simulink model "LinearADPSimullink_R2014b"  (R2014b)
settings: Solver=ode45  StartTime=0.0  StopTime=10  MaxStep=0.0001  RelTol=1e-3
undefined symbols (not defined in the file): rank
libraries: simulink x4
settings Model: Creator=Yuri  LastModifiedBy=yujiang
settings SolverCC: ZeroCrossControl=EnableAll  ZeroCrossAlgorithm=Adaptive
settings DebuggingCC: AlgebraicLoopMsg=none  MultiTaskDSMMsg=none  FrameProcessingCompatibilityMsg=error
settings RTWCC: GenCodeOnly=on

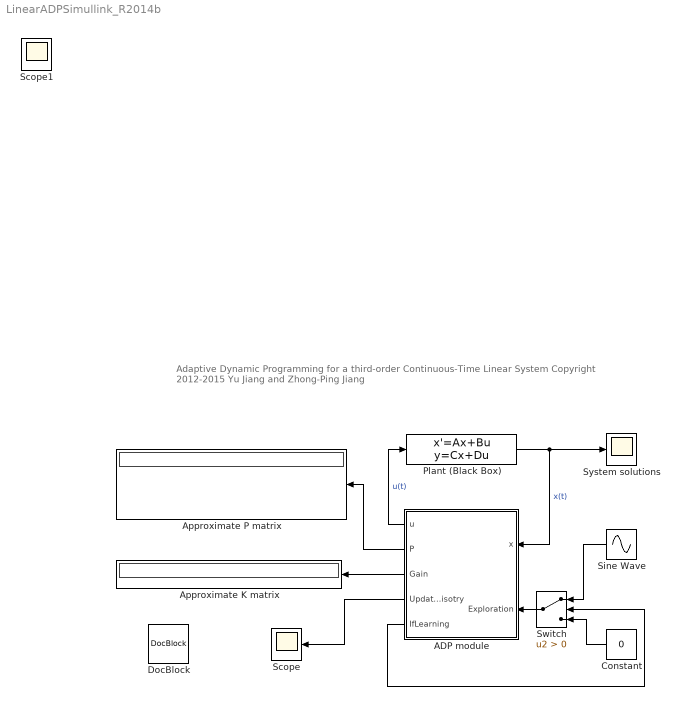
== system LinearADPSimullink_R2014b ==
  note: Adaptive Dynamic Programming for a third-order Continuous-Time Linear System
      |
      | Copyright 2012-2015 Yu Jiang and Zhong-Ping Jiang
  ADP module : Subsystem  mask{K=[0,0,0], Q=eye(3), R=1, dT=0.1, epsilon=.00005}
      mask prompts: K "Initial Gain K (e.g., [0,0])"; Q "Weight Matrix Q (e.g., eye(2))"; R "Weight R (e.g., 1)"; dT "Linearning Interval (e.g., 0.01)"; epsilon "Threshold (e.g., 0.00001)"
  Approximate K matrix : Display
  Approximate P matrix : Display
  Constant : Constant  Value=0
  DocBlock : simulink/Model-Wide Utilities/DocBlock  DocumentType=Text
      content=|
      | %To verify the results, try:
      |
      | A = [0 1 0; 0 0 1;-0.1 -0.5 -0.7];
      | B = [0;0;1];
      | Q = eye(3);
      | R = 1;
      |
      | [Popt,~,Kopt] = care(A,B,Q,R)
  Plant (Black Box) : StateSpace  A=[0 1 0; 0 0 1;-0.1 -0.5 -0.7]  B=[0;0;1]  C=eye(3)  D=zeros(3,1)  X0=[10;-10;15]
  Scope : Scope
      settings: SaveName=ScopeData2
  Sine Wave : Sin  Amplitude=2  Frequency=10  SampleTime=0.0001
  Switch : Switch  Criteria=u2 > Threshold  SampleTime=0.0001
  "System solutions " : Scope
      settings: ShowLegends=on  TimeRange=10  YMin=-10  YMax=20
  Scope1 : Scope
      settings: SaveName=ScopeData2
  wires:
  Plant (Black Box)/1 -> ADP module/1(x), "System solutions "/1  "x(t)"
  ADP module/1(u) -> Plant (Black Box)/1  "u(t)"
  ADP module/2("P ") -> Approximate P matrix/1
  ADP module/3(Gain) -> Approximate K matrix/1
  ADP module/4(UpdateHisotry) -> Scope/1
  Sine Wave/1 -> Switch/1
  Switch/1 -> ADP module/2(Exploration)
  ADP module/5(IfLearning) -> Switch/2
  Constant/1 -> Switch/3

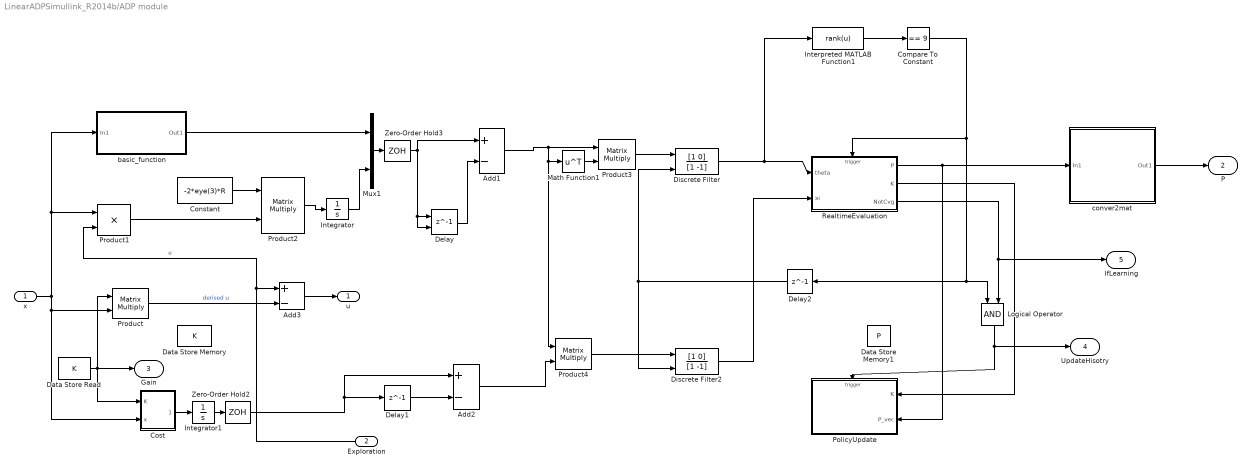
== system LinearADPSimullink_R2014b/ADP module ==
  x : Inport  PortDimensions=3
  Exploration : Inport  Port=2
  Add1 : Sum  Inputs=+-
  Add2 : Sum  Inputs=+-
  Add3 : Sum  Inputs=+-
  Compare To Constant : simulink/Logic and Bit Operations/Compare To Constant  relop===  const=9  OutDataTypeStr=boolean
  Constant : Constant  Value=-2*eye(3)*R  VectorParams1D=off
  Cost : Subsystem
  Data Store Memory : DataStoreMemory  Priority=1  DataStoreName=K  InitialValue=K  VectorParams1D=off  Dimensions=[1,3]
  Data Store Memory1 : DataStoreMemory  DataStoreName=P  InitialValue=-1*ones(6,1)
  Data Store Read : DataStoreRead  DataStoreName=K  SampleTime=0
  Delay : Delay  DelayLength=1  InitialConditionSource=Input port  InitialCondition=0  SampleTime=dT
      settings: InputPortMap=u0,p4
  Delay1 : Delay  DelayLength=1  InitialCondition=0  SampleTime=dT
  Delay2 : Delay  DelayLength=1  InitialCondition=0  SampleTime=dT
  Discrete Filter : DiscreteFilter  Numerator=[1 0]  Denominator=[1 -1]  ExternalReset=Rising  FilterStructure=Direct form I  SampleTime=dT  NumAccumDataTypeStr=Inherit: Same as product output  OutDataTypeStr=Inherit: Same as input
      settings: InputPortMap=u0,r7
  Discrete Filter2 : DiscreteFilter  Numerator=[1 0]  Denominator=[1 -1]  ExternalReset=Rising  FilterStructure=Direct form I  SampleTime=dT  NumAccumDataTypeStr=Inherit: Same as product output  OutDataTypeStr=Inherit: Same as input
      settings: InputPortMap=u0,r7
  Integrator : Integrator
  Integrator1 : Integrator
  Interpreted MATLAB Function1 : MATLABFcn  MATLABFcn=rank(u)  OutputDimensions=1
  Logical Operator : Logic  AllPortsSameDT=off  OutDataTypeStr=boolean
  Math Function1 : Math  Operator=transpose  SaturateOnIntegerOverflow=on
  Mux1 : Mux  Inputs=2
  PolicyUpdate : Subsystem
  Product{,2..4} (4 alike) : Product  Multiplication=Matrix(*)
  Product1 : Product
  RealtimeEvaluation : Subsystem
  Zero-Order Hold2 : ZeroOrderHold  SampleTime=dT
  Zero-Order Hold3 : ZeroOrderHold  SampleTime=dT
  basic_function : Subsystem
  conver2mat : Subsystem
  u : Outport
  "P " : Outport  Port=2
  Gain : Outport  Port=3
  UpdateHisotry : Outport  Port=4
  IfLearning : Outport  Port=5
  wires:
  RealtimeEvaluation/3(NotCvg) -> Logical Operator/2, IfLearning/1
  Exploration/1 -> Add3/1, Product1/2  "e"
  Logical Operator/1 -> PolicyUpdate/Trigger, UpdateHisotry/1
  Compare To Constant/1 -> Delay2/1, Logical Operator/1, RealtimeEvaluation/Trigger
  Add1/1 -> Product3/1, Math Function1/1, Product4/1
  Delay2/1 -> Discrete Filter2/2, Discrete Filter/2
  Zero-Order Hold2/1 -> Delay1/1, Add2/1
  Mux1/1 -> Zero-Order Hold3/1
  Discrete Filter2/1 -> RealtimeEvaluation/2(xi)
  Discrete Filter/1 -> Interpreted MATLAB Function1/1, RealtimeEvaluation/1(theta)
  Product4/1 -> Discrete Filter2/1
  Add2/1 -> Product4/2
  Product3/1 -> Discrete Filter/1
  Math Function1/1 -> Product3/2
  Add3/1 -> u/1
  Delay1/1 -> Add2/2
  Integrator1/1 -> Zero-Order Hold2/1
  Cost/1(r(x,uk)) -> Integrator1/1
  Delay/1 -> Add1/2
  Zero-Order Hold3/1 -> Add1/1, Delay/1, Delay/2
  Integrator/1 -> Mux1/2
  Product2/1 -> Integrator/1
  Constant/1 -> Product2/1
  Product1/1 -> Product2/2
  Data Store Read/1 -> Product/1, Cost/1(K), Gain/1
  Product/1 -> Add3/2  "derised u"
  x/1 -> basic_function/1(In1), Product1/1, Product/2, Cost/2(x)
  RealtimeEvaluation/1(P) -> PolicyUpdate/2("P_vec "), conver2mat/1(In1)
  RealtimeEvaluation/2(K) -> PolicyUpdate/1(K)
  Interpreted MATLAB Function1/1 -> Compare To Constant/1
  basic_function/1(Out1) -> Mux1/1
  conver2mat/1(Out1) -> "P "/1

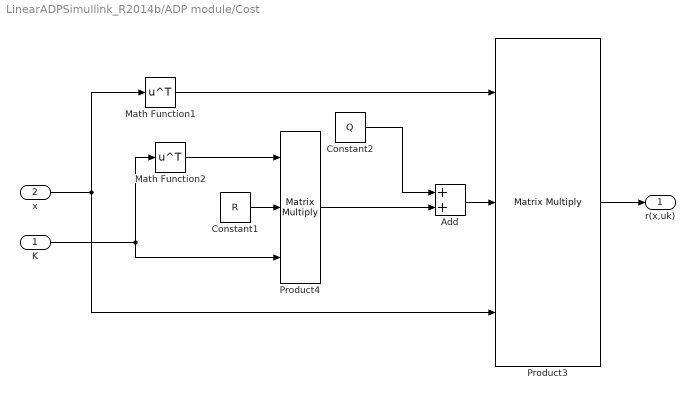
== system LinearADPSimullink_R2014b/ADP module/Cost ==
  K : Inport
  x : Inport  Port=2  PortDimensions=3
  Add : Sum
  Constant1 : Constant  Value=R
  Constant2 : Constant  Value=Q
  Math Function1 : Math  Operator=transpose  SaturateOnIntegerOverflow=on
  Math Function2 : Math  Operator=transpose  SaturateOnIntegerOverflow=on
  Product3 : Product  Inputs=3  Multiplication=Matrix(*)
  Product4 : Product  Inputs=3  Multiplication=Matrix(*)
  r(x,uk) : Outport
  wires:
  Math Function2/1 -> Product4/1
  Constant1/1 -> Product4/2
  K/1 -> Product4/3, Math Function2/1
  Constant2/1 -> Add/1
  Product3/1 -> r(x,uk)/1
  Math Function1/1 -> Product3/1
  Product4/1 -> Add/2
  x/1 -> Product3/3, Math Function1/1
  Add/1 -> Product3/2

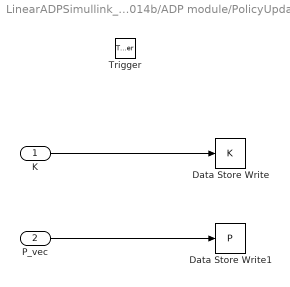
== system LinearADPSimullink_R2014b/ADP module/PolicyUpdate ==
  K : Inport  OutDataTypeStr=double  PortDimensions=[1,3]
  "P_vec " : Inport  Port=2  PortDimensions=6
  Trigger : TriggerPort  OutputDataType=double  PortDimensions=1
  Data Store Write : DataStoreWrite  DataStoreName=K
  Data Store Write1 : DataStoreWrite  DataStoreName=P
  wires:
  "P_vec "/1 -> Data Store Write1/1
  K/1 -> Data Store Write/1

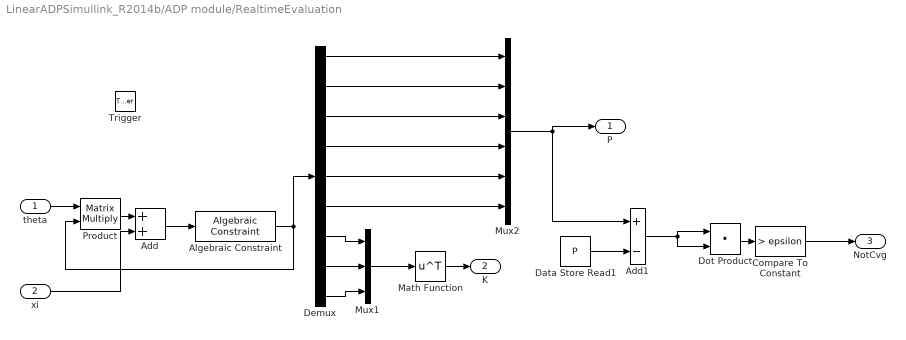
== system LinearADPSimullink_R2014b/ADP module/RealtimeEvaluation ==
  theta : Inport
  xi : Inport  Port=2
  Trigger : TriggerPort  OutputDataType=double  PortDimensions=1
  Add : Sum
  Add1 : Sum  Inputs=+-
  Algebraic Constraint : simulink/Math Operations/Algebraic Constraint  z0=zeros(9,1)
  Compare To Constant : simulink/Logic and Bit Operations/Compare To Constant  relop=>  const=epsilon  OutDataTypeStr=boolean
  Data Store Read1 : DataStoreRead  DataStoreName=P
  Demux : Demux  Outputs=9
  Dot Product : DotProduct  InputSameDT=on  OutDataTypeStr=Inherit: Inherit via internal rule
  Math Function : Math  Operator=transpose  SaturateOnIntegerOverflow=on
  Mux1 : Mux  Inputs=3
  Mux2 : Mux  Inputs=6
  Product : Product  Multiplication=Matrix(*)  OutDataTypeStr=double
  P : Outport  OutDataTypeStr=double  PortDimensions=6  InitialOutput=zeros(6,1)
  K : Outport  Port=2  PortDimensions=[1,3]  InitialOutput=K
  NotCvg : Outport  Port=3  PortDimensions=1  InitialOutput=1
  wires:
  Compare To Constant/1 -> NotCvg/1
  Mux2/1 -> Add1/1, P/1
  Dot Product/1 -> Compare To Constant/1
  Add1/1 -> Dot Product/1, Dot Product/2
  Data Store Read1/1 -> Add1/2
  Product/1 -> Add/1
  theta/1 -> Product/1
  Algebraic Constraint/1 -> Product/2, Demux/1
  Add/1 -> Algebraic Constraint/1
  xi/1 -> Add/2
  Math Function/1 -> K/1
  Mux1/1 -> Math Function/1
  Demux/7 -> Mux1/1
  Demux/8 -> Mux1/2
  Demux/9 -> Mux1/3
  Demux/1 -> Mux2/1
  Demux/2 -> Mux2/2
  Demux/3 -> Mux2/3
  Demux/4 -> Mux2/4
  Demux/5 -> Mux2/5
  Demux/6 -> Mux2/6

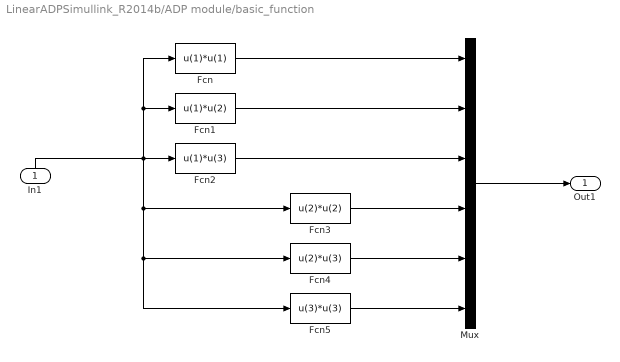
== system LinearADPSimullink_R2014b/ADP module/basic_function ==
  In1 : Inport
  Fcn : Fcn  Expr=u(1)*u(1)
  Fcn1 : Fcn  Expr=u(1)*u(2)
  Fcn2 : Fcn  Expr=u(1)*u(3)
  Fcn3 : Fcn  Expr=u(2)*u(2)
  Fcn4 : Fcn  Expr=u(2)*u(3)
  Fcn5 : Fcn  Expr=u(3)*u(3)
  Mux : Mux  Inputs=6
  Out1 : Outport  PortDimensions=6
  wires:
  Mux/1 -> Out1/1
  Fcn2/1 -> Mux/3
  Fcn/1 -> Mux/1
  Fcn1/1 -> Mux/2
  Fcn3/1 -> Mux/4
  Fcn4/1 -> Mux/5
  Fcn5/1 -> Mux/6
  In1/1 -> Fcn1/1, Fcn/1, Fcn3/1, Fcn5/1, Fcn4/1, Fcn2/1

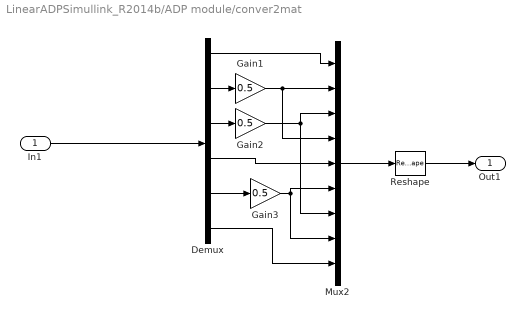
== system LinearADPSimullink_R2014b/ADP module/conver2mat ==
  In1 : Inport
  Demux : Demux  Outputs=6
  Gain1 : Gain  Gain=0.5
  Gain2 : Gain  Gain=0.5
  Gain3 : Gain  Gain=0.5
  Mux2 : Mux  Inputs=9
  Reshape : Reshape  OutputDimensionality=Customize  OutputDimensions=[3,3]
  Out1 : Outport
  wires:
  In1/1 -> Demux/1
  Demux/2 -> Gain1/1
  Demux/3 -> Gain2/1
  Mux2/1 -> Reshape/1
  Gain3/1 -> Mux2/8, Mux2/6
  Reshape/1 -> Out1/1
  Demux/5 -> Gain3/1
  Gain2/1 -> Mux2/7, Mux2/3
  Gain1/1 -> Mux2/4, Mux2/2
  Demux/1 -> Mux2/1
  Demux/4 -> Mux2/5
  Demux/6 -> Mux2/9
